simulink model "MBSE_Project_SeatBeltRemainderalternate"  (R2020b)
settings: Solver=VariableStepAuto  StartTime=0.0  StopTime=inf  RelTol=1e-3
settings Model: Creator=99003747  LastModifiedBy=99003747

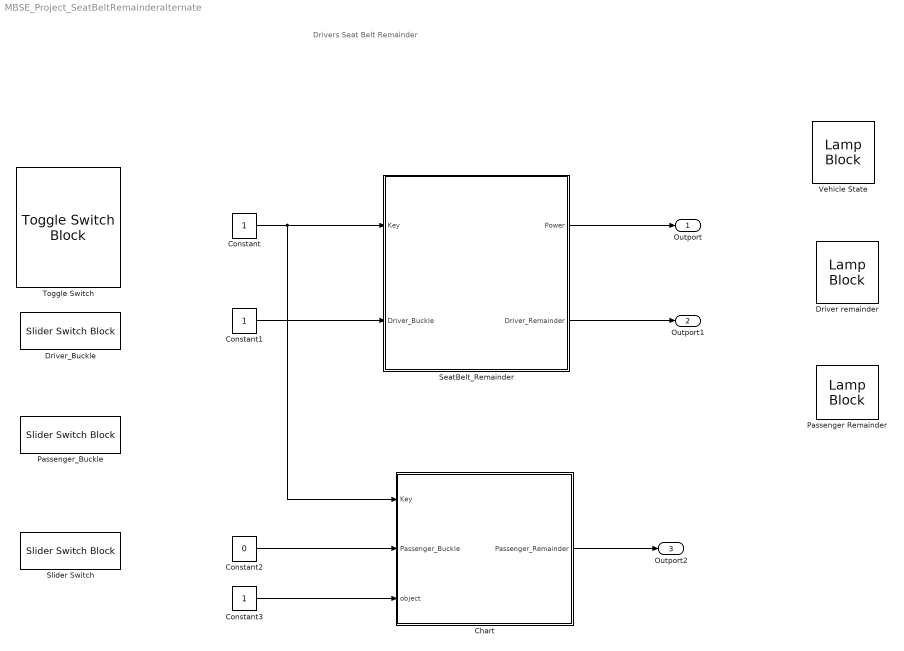
== system MBSE_Project_SeatBeltRemainderalternate ==
  note: Drivers Seat Belt Remainder
  " Passenger_Buckle" : SliderSwitchBlock
      settings: Values={{'Off', 'On'}, [0 1]}
  Chart : Stateflow chart  TreatAsAtomicUnit=on
  Constant : Constant
  Constant1 : Constant
  Constant2 : Constant  Value=0
  Constant3 : Constant
  Driver remainder : LampBlock
  Driver_Buckle : SliderSwitchBlock
      settings: Values={{'Off', 'On'}, [0 1]}
  Passenger Remainder : LampBlock
  SeatBelt_Remainder : Stateflow chart  TreatAsAtomicUnit=on
  Slider Switch : SliderSwitchBlock
      settings: Values={{'Off', 'On'}, [0 1]}
  Toggle Switch : ToggleSwitchBlock
      settings: Values={{'Off', 'On'}, [0 1]}
  Vehicle State : LampBlock
  Outport : Outport
  Outport1 : Outport  Port=2
  Outport2 : Outport  Port=3
  wires:
  Constant/1 -> Chart/1(Key), SeatBelt_Remainder/1(Key)
  Constant1/1 -> SeatBelt_Remainder/2(Driver_Buckle)
  SeatBelt_Remainder/1(Power) -> Outport/1
  SeatBelt_Remainder/2(Driver_Remainder) -> Outport1/1
  Chart/1(Passenger_Remainder) -> Outport2/1
  Constant2/1 -> Chart/2(Passenger_Buckle)
  Constant3/1 -> Chart/3(object)

== stateflow chart MBSE_Project_SeatBeltRemainderalternate/SeatBelt_Remainder ==
  state Indicator
    entry:
    Power=1;
    Driver_Remainder=1 ;
  state VehicleOff
    entry:
    Power=0;
    Driver_Remainder=0;
  state SeatBeltBuckled
    entry:
    Driver_Remainder=0;
  SeatBeltBuckled -> VehicleOff [order 2] : [Key == 0]
  (default) -> VehicleOff
  Indicator -> SeatBeltBuckled [order 1] : [Driver_Buckle==1]
  Indicator -> VehicleOff [order 2] : after(5,sec) [Key==0]
  SeatBeltBuckled -> Indicator [order 1] : [Driver_Buckle == 0]
  VehicleOff -> Indicator : [Key==1 ]
  data: Power output; Key input =0; Driver_Buckle input; Driver_Remainder output

== stateflow chart MBSE_Project_SeatBeltRemainderalternate/Chart ==
  state passenger_state
    entry:
    Power=0;
    Passenger_Remainder=0;
  state remainder
    entry:
    Passenger_Remainder = 0;
  state object_detection
    entry:
    Power=1;
    Passenger_Remainder=0;
  state Object
    entry:
    Passenger_Remainder =1;
  remainder -> passenger_state [order 1] : [Key == 0]
  Object -> passenger_state [order 3] : [Key == 0]
  (default) -> passenger_state
  Object -> remainder [order 1] : [Passenger_Buckle == 1]
  object_detection -> passenger_state [order 1] : [Key == 0 ]
  object_detection -> Object [order 2] : [object == 1]
  remainder -> Object [order 2] : [Passenger_Buckle == 0]
  passenger_state -> object_detection : [ Key== 1 ]
  Object -> object_detection [order 2] : [object == 0]
  data: Key input; Passenger_Buckle input; Passenger_Remainder output; object input; Power local
